simulink model "pendule_inv_etu"  (R2019a)
settings: Solver=ode23t  StartTime=0.0  StopTime=1000  RelTol=1e-3
values from neighbouring files (symbols this model uses):
  g = 9.81    [simu_pendule_inv_capteur_etu.m]
  K = [10 1]    [simu_pendule_inv_capteur_etu.m]
  l = 10    [simu_pendule_inv_capteur_etu.m]
  ue = 0    [simu_pendule_inv_capteur_etu.m]
  xe = [0 0]'    [simu_pendule_inv_capteur_etu.m]
libraries: simulink x1
settings Model: Creator=nfoin  LastModifiedBy=nfoin

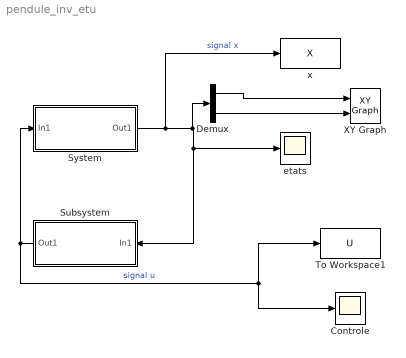
== system pendule_inv_etu ==
  Controle : Scope
  Demux : Demux  Outputs=2
  Subsystem : Subsystem
  System : Subsystem
  To Workspace1 : ToWorkspace  VariableName=U  SaveFormat=Timeseries  SampleTime=-1
  XY Graph : simulink/Sinks/XY Graph  xmin=-1  xmax=1  ymin=-1  ymax=1  st=-1
  etats : Scope
  x : ToWorkspace  VariableName=X  SaveFormat=Timeseries  SampleTime=-1
  wires:
  System/1(Out1) -> x/1, Demux/1, Subsystem/1(In1), etats/1  "signal x"
  Subsystem/1(Out1) -> System/1(In1), To Workspace1/1, Controle/1  "signal u"
  Demux/1 -> XY Graph/1
  Demux/2 -> XY Graph/2

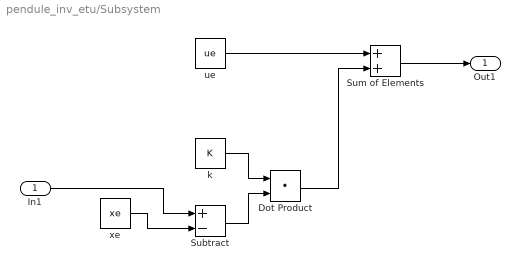
== system pendule_inv_etu/Subsystem ==
  In1 : Inport
  Dot Product : DotProduct  InputSameDT=on  OutDataTypeStr=Inherit: Inherit via internal rule
  Subtract : Sum  Inputs=+-
  Sum of Elements : Sum
  k : Constant  Value=K
  ue : Constant  Value=ue
  xe : Constant  Value=xe
  Out1 : Outport
  wires:
  ue/1 -> Sum of Elements/1
  In1/1 -> Subtract/1
  xe/1 -> Subtract/2
  k/1 -> Dot Product/1
  Subtract/1 -> Dot Product/2
  Dot Product/1 -> Sum of Elements/2
  Sum of Elements/1 -> Out1/1

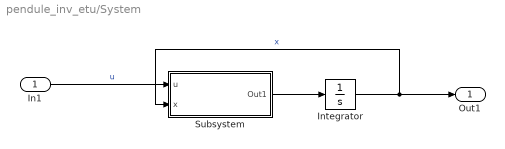
== system pendule_inv_etu/System ==
  In1 : Inport
  Integrator : Integrator  InitialCondition=-1
  Subsystem : Subsystem
  Out1 : Outport
  wires:
  In1/1 -> Subsystem/1(u)  "u"
  Subsystem/1(Out1) -> Integrator/1
  Integrator/1 -> Subsystem/2(x), Out1/1  "x"

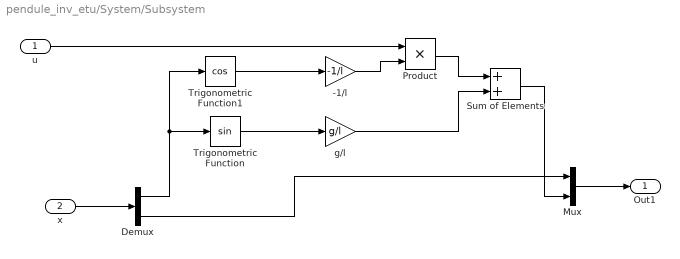
== system pendule_inv_etu/System/Subsystem ==
  u : Inport
  x : Inport  Port=2
  -1/l : Gain  Gain=-1/l
  Demux : Demux  Outputs=2
  Mux : Mux  Inputs=2
  Product : Product
  Sum of Elements : Sum
  Trigonometric Function : Trigonometry
  Trigonometric Function1 : Trigonometry  Operator=cos
  g/l : Gain  Gain=g/l
  Out1 : Outport
  wires:
  x/1 -> Demux/1
  Demux/1 -> Trigonometric Function1/1, Trigonometric Function/1
  Mux/1 -> Out1/1
  Trigonometric Function/1 -> g/l/1
  Demux/2 -> Mux/1
  Trigonometric Function1/1 -> -1/l/1
  -1/l/1 -> Product/2
  Product/1 -> Sum of Elements/1
  g/l/1 -> Sum of Elements/2
  u/1 -> Product/1
  Sum of Elements/1 -> Mux/2
